simulink model "rejz2"  (R2021a)
settings: Solver=VariableStepAuto  StartTime=0.0  StopTime=10.0  RelTol=1e-3
values from neighbouring files (symbols this model uses):
  R = R1v    [apr27.m]
  S = sol(3:end)'    [apr27.m]
  T = Bmv*Ao    [apr27.m]
  Ts = 0.2    [apr27.m]
libraries: cstblocks x3
settings Model: Creator=Peti  LastModifiedBy=Peti

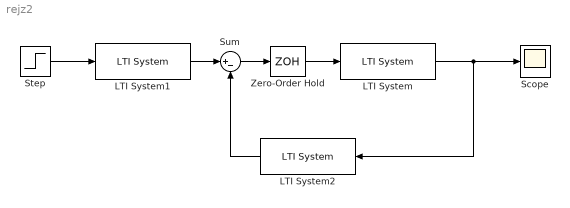
== system rejz2 ==
  LTI System : cstblocks/LTI System  sys=W  IC=[]
  LTI System1 : cstblocks/LTI System  sys=tf(T,R,Ts)  IC=[]
  LTI System2 : cstblocks/LTI System  sys=tf(S,R,Ts)  IC=[]
  Scope : Scope
  Step : Step  SampleTime=0
  Sum : Sum  Inputs=|+-
  Zero-Order Hold : ZeroOrderHold  SampleTime=-1
  wires:
  LTI System1/1 -> Sum/1
  Zero-Order Hold/1 -> LTI System/1
  Sum/1 -> Zero-Order Hold/1
  LTI System/1 -> LTI System2/1, Scope/1
  LTI System2/1 -> Sum/2
  Step/1 -> LTI System1/1
